simulink model "simulink8"  (R2025b)
settings: Solver=ode45  StartTime=0.0  StopTime=15.0  MaxStep=0.02  MinStep=0.01  RelTol=1e-3
settings Model: Creator=mizula  LastModifiedBy=mizula
settings SolverCC: InitialStep=0.01

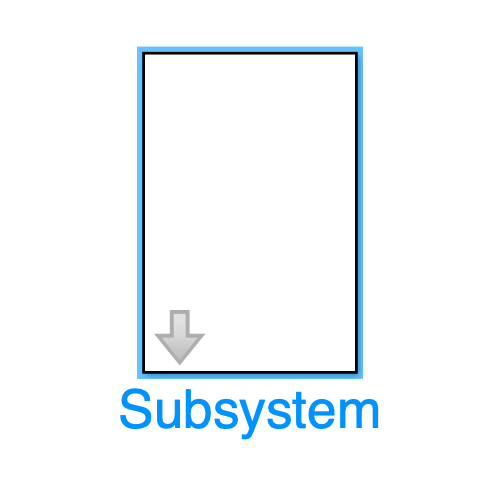
[thumbnail: Simulink's stored preview of the top-level diagram]
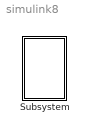
== system simulink8 ==
  Subsystem : Subsystem  mask{g=9.81, k=1, m=2, l=4, x0=-1, y0=-1, xi=[-1 1 1], yi=[1 1 -1], di=[0.1 0.1 0.1], ai=[1 -1 1.5]}

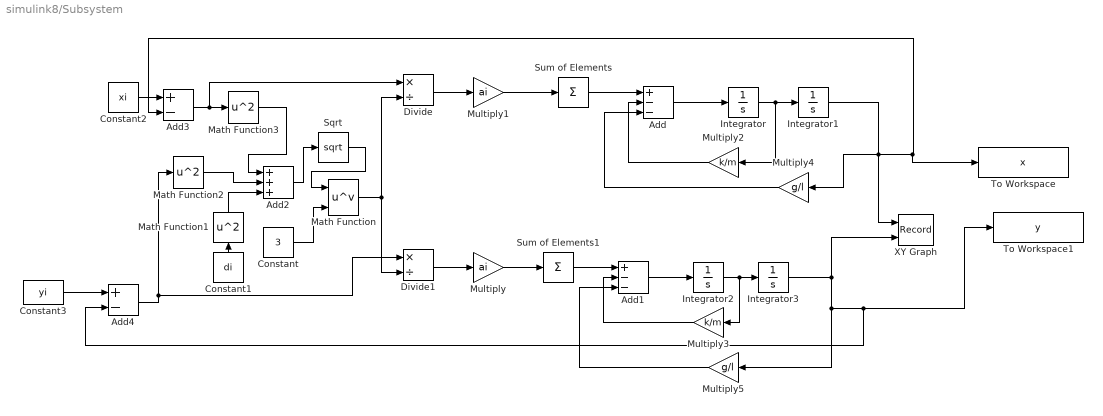
== system simulink8/Subsystem ==
  Add : Sum  Inputs=+--
  Add1 : Sum  Inputs=+--
  Add2 : Sum  Inputs=+++
  Add3 : Sum  Inputs=+-
  Add4 : Sum  Inputs=+-
  Constant : Constant  Value=3
  Constant1 : Constant  Value=di
  Constant2 : Constant  Value=xi
  Constant3 : Constant  Value=yi
  Divide : Product  Inputs=*/
  Divide1 : Product  Inputs=*/
  Integrator : Integrator
  Integrator1 : Integrator  InitialCondition=x0
  Integrator2 : Integrator
  Integrator3 : Integrator  InitialCondition=y0
  Math Function : Math  Operator=pow  SignedPower=on
  Math Function1 : Math  Operator=square
  Math Function2 : Math  Operator=square
  Math Function3 : Math  Operator=square
  Multiply : Gain  Gain=ai
  Multiply1 : Gain  Gain=ai
  Multiply2 : Gain  Gain=k/m
  Multiply3 : Gain  Gain=k/m
  Multiply4 : Gain  Gain=g/l
  Multiply5 : Gain  Gain=g/l
  Sqrt : Sqrt
  Sum of Elements : Sum  Inputs=1
  Sum of Elements1 : Sum  Inputs=1
  To Workspace : ToWorkspace  VariableName=x  SaveFormat=Timeseries  SampleTime=-1
  To Workspace1 : ToWorkspace  VariableName=y  SaveFormat=Timeseries  SampleTime=-1
  XY Graph : Record  NumPorts=2.0  FileSettingsInternal="{\"entries\":[{\"content\":{\"excelSettings\":{\"content\":{},\"type\":\"Streamout.ExcelSettings\"},\"parquetSettings\":{\"content\":{},\"type\":\"Streamout.ParquetSettings\"}},\"type\":\"Streamout.FileSettingStorage\",\"uuid\":\"\"}],\"packageUris\":[\"http:\\/\\/schema.mathworks.com\\/mf0\\/streamout_blocks\\/R2020a\"],\"version\":\"1.0\"}"  FrameSettings=[0, 0]  Layout=[1 1]  SignalsInternal="{\"entries\":[{\"content\":{\"signals\":[{\"content\":{\"blockPath\":[],\"dimensions\":[1],\"domain\":\"\",\"lineColor\":\"#a2142f\",\"plots\":[ 1 ],\"port\":1,\"sid\":[\"\"],\"signalID\":1,\"signalName\":\"Integrator1\"},\"type\":\"RecordBlkView.Signal\",\"uuid\":\"\"},{\"content\":{\"blockPath\":[],\"dimensions\":[1],\"domain\":\"\",\"lineColor\":\"#139fff\",\"plots\":[ 1 ],\"port\":2,\"sid\":[\"\"],\"signalID\":2,\"signalName\":\"Integrator3\"},\"type\":\"RecordBlkView.Signal\",\"uuid\":\"\"}]},\"type\":\"RecordBlkView.InputSignals\",\"uuid\":\"\"}],\"packageUris\":[\"http:\\/\\/schema.mathworks.com\\/mf0\\/streamout_blocks\\/R2020a\"],\"version\":\"1.0\"}"  VisualizationBindings="{\"xyplotplugin\":{\"info\":[{\"series\":[{\"bindingParametersList\":[{\"parameter\":\"X-Axis\",\"signalID\":1,\"signalName\":\"Integrator1\"},{\"parameter\":\"Y-Axis\",\"signalID\":2,\"signalName\":\"Integrator3\"}],\"seriesID\":0}],\"subplotID\":1}]}}"  CompatibilityTag=XY
  wires:
  Constant1/1 -> Math Function1/1
  Add1/1 -> Integrator2/1
  Math Function2/1 -> Add2/2
  Multiply1/1 -> Sum of Elements/1
  Multiply4/1 -> Add/3
  Constant/1 -> Math Function/2
  Add4/1 -> Math Function2/1, Divide1/1
  Integrator/1 -> Multiply2/1, Integrator1/1
  Multiply3/1 -> Add1/2
  Add/1 -> Integrator/1
  Math Function3/1 -> Add2/1
  Integrator2/1 -> Multiply3/1, Integrator3/1
  Integrator3/1 -> XY Graph/2, To Workspace1/1, Add4/2, Multiply5/1
  Multiply/1 -> Sum of Elements1/1
  Math Function/1 -> Divide/2, Divide1/2
  Multiply5/1 -> Add1/3
  Divide/1 -> Multiply1/1
  Add3/1 -> Divide/1, Math Function3/1
  Sum of Elements1/1 -> Add1/1
  Sum of Elements/1 -> Add/1
  Constant3/1 -> Add4/1
  Divide1/1 -> Multiply/1
  Integrator1/1 -> XY Graph/1, To Workspace/1, Add3/2, Multiply4/1
  Constant2/1 -> Add3/1
  Math Function1/1 -> Add2/3
  Multiply2/1 -> Add/2
  Add2/1 -> Sqrt/1
  Sqrt/1 -> Math Function/1
